simulink model "Controller_Block"  (R2022b)
settings: Solver=VariableStepAuto  StartTime=0.0  StopTime=10.0  RelTol=1e-3
undefined symbols (not defined in the file): G
settings Model: Creator=Akash  LastModifiedBy=Akash

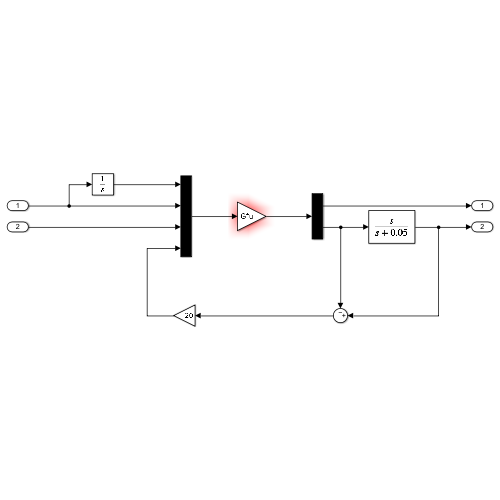
[thumbnail: Simulink's stored preview of the top-level diagram]
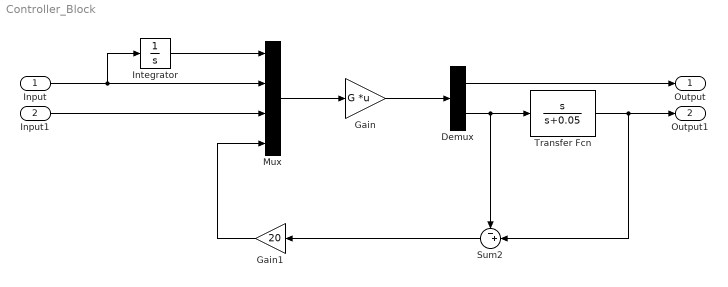
== system Controller_Block ==
  Input : Inport
  Input1 : Inport  Port=2
  Demux : Demux  Outputs=2
  Gain : Gain  Gain=G  Multiplication=Matrix(K*u)
  Gain1 : Gain  Gain=20
  Integrator : Integrator
  Mux : Mux
  Sum2 : Sum  Inputs=-+|
  Transfer Fcn : TransferFcn  Numerator=[1 0]  Denominator=[1 0.05]
  Output : Outport
  Output1 : Outport  Port=2
  wires:
  Mux/1 -> Gain/1
  Integrator/1 -> Mux/1
  Input/1 -> Integrator/1, Mux/2
  Input1/1 -> Mux/3
  Gain1/1 -> Mux/4
  Sum2/1 -> Gain1/1
  Gain/1 -> Demux/1
  Demux/2 -> Sum2/1, Transfer Fcn/1
  Demux/1 -> Output/1
  Transfer Fcn/1 -> Sum2/2, Output1/1
